simulink model "Copy_of_MPC_control"  (R2018a)
settings: Solver=FixedStepAuto  StartTime=0  StopTime=Tend  FixedStep=0.001  RelTol=5e-3
model workspace (MAT data in the model file):
  A_mu = 10
  B_reff = 8.386
  Cz = 7766.25
  DCT_Param : struct (value not decoded)
  D_reff = 0.25826
  Downshift_Speeds = [9.5625 12.9375 16.3125 19.6875 23.0625 26.4375 29.8125 33.1875 36.5625 39.9375 43.3125 46.6875 ... (28 elements, 4x7)]
  Pedal_Positions = [0.1 0.4 0.5 0.9]
  SUS : struct (value not decoded)
  Upshift_Speeds = [12.9375 16.3125 19.6875 33 26.4375 29.8125 33.1875 52.5 39.9375 43.3125 46.6875 77.25 ... (28 elements, 4x7)]
  VEH : struct (value not decoded)
  V_o = 16.7
  V_xlow = 1
  WH : struct (value not decoded)
  a = 1.4
  alpha_max = 1.5
  alpha_min = -1.5
  b = 1.8
  c_zo = 209651
  epsilon = 0.1
  h = 0.134
  path : struct (value not decoded)
  pio = 220000
  q_Fcx = 0
  q_Fz2 = 15.4
  q_Fzy = 0
  q_reo = 0.9974
  q_sx1 = -0.007764
  q_sx10 = 0.2824
  q_sx11 = 5.349
  q_sx12 = 0
  q_sx13 = 0
  q_sx14 = 0
  q_sx2 = 1.1915
  q_sx3 = 0.013948
  q_sx4 = 4.912
  q_sx5 = 1.02
  q_sx6 = 22.83
  q_sx7 = 0.7104
  q_sx8 = -0.023393
  q_sx9 = 0.6581
  q_sy1 = 0.00702
  q_sy2 = 0
  q_sy3 = 0.001515
  q_sy4 = 8.514e-05
  q_sy5 = 0
  q_sy6 = 0
  q_sy7 = 0.9008
  q_sy8 = -0.4089
  q_v1 = 0.0007742
  q_v2 = 0.04667
  r_Bx1 = 12.531
  r_Bx2 = 9.532
  r_Bx3 = 0
  r_By1 = 10.615
  r_By2 = 7.705
  r_By3 = 3.433e-06
  r_By4 = 0
  r_Cx1 = 1.019
  r_Cy1 = 1.0585
  r_Ex1 = -0.4487
  r_Ex2 = -0.4726
  r_Ey1 = 0.3132
  r_Ey2 = 7.63e-06
  r_Hx1 = 0.0002374
  r_Hy1 = 0.011646
  r_Hy2 = 7.63e-06
  r_Vy1 = 0.05654
  r_Vy2 = 7.63e-06
  r_Vy3 = 0
  r_Vy4 = 99.9
  r_Vy5 = 2
  r_Vy6 = 15.814
  r_o = 0.3135
  vehWidth = 2
  w = 1
symbols that are objects in the model workspace (value not decoded): VEH
undefined symbols (not defined in the file): C_Brake, C_Final, C_Front, C_Front_1, C_Front_2, C_Middle, C_out_Brake, C_out_Final, C_out_Front, C_out_Front_1, C_out_Front_2, C_out_Middle, Co, Cok_Brake, Cok_Final, Cok_Front_1, Cok_Front_2, Cok_Middle, Cso, D_out_Brake, D_out_Final, D_out_Front, D_out_Front_1, D_out_Front_2, D_out_Middle, Earlytochange, Earlytochange2, F, F_Brake, F_Final, F_Front, F_Front_1, F_Front_2, F_Middle, Fs, G_Brake, G_Final, G_Front_1, G_Front_2, G_Middle, G_sys_Brake, G_sys_Final, G_sys_Front, G_sys_Front_1, G_sys_Front_2, G_sys_Middle, Gd, Gd_Brake, Gd_Final, Gd_Front, Gd_Front_1, Gd_Front_2, Gd_Middle, Go, Gsd, Gso, H_Brake, H_Final, H_Front_1, H_Front_2 ... (+60)
libraries: simulink x10, sim3dlib x4, autolibutils x2, vehdynlibviscommon x2
(part 3 of 8)

== system Copy_of_MPC_control/all_system/Visualization1 ==
  note: Driver Commands
  note: Vehicle Response
  Cntrl : Inport
  VehFdbk : Inport  Port=2
  3D Engine : Subsystem  Variant=on  OverrideUsingVariant=0  mask(3D Engine){engine3D=Disabled, SceneDesc=Straight road, dt3D=.03}
      mask prompts: engine3D "3D Engine"; SceneDesc "Scene Description:"; dt3D "Engine frame rate, dt3D [s]:"
      mask help: This subsystem contains the interface blocks which permit the display of the vehicle in 3D virtual environment. Enable it to view the simulation progress, disable it to inhibit the display.
      mask init: same as Copy_of_MPC_control/Visualization/3D Engine
      settings: AttributesFormatString=%<engine3D>
      mask Help: eval('vdynblkshelp(''vdynblksscenecameraray'')');
      mask TypeOptions engine3D: Enabled | Disabled
      mask Callback engine3D:
      | switch get_param(gcb,'engine3D')
      |     case 'Disabled'
      |         set_param(gcb,'OverrideUsingVariant','0')
      |     case 'Enabled'
      |        set_param(gcb,'OverrideUsingVariant','1')
      |     otherwise
      |        set_param(gcb,'OverrideUsingVariant','0')
      | end
      mask TypeOptions SceneDesc:
      | 3D Engine/Simulation 3D Engine
      | 1/SceneDesc
      mask Display: disp('3D Engine')
  Acceleration Cmd : Subsystem  DialogController=hmiCreateDDGDialog  IsWebBlock=on  mask(MWDashboardBlock){webBlockId=2ec56b20-76c2-4aac-ab3d-2dd24ca42fe8, webBlockType=lineargauge, ShowInLibBrowser=on, ShowInitialText=on, HMISrcModelName=MPC_control}
      mask prompts: webBlockId "WebBlock Id"; webBlockType "WebBlock Type"; HMISrcModelName "Source Model"
      mask help: SimulinkHMI:dialogs:LinearGaugeDialogDesc
      mask Help: helpview([docroot '/mapfiles/simulink.map'], 'hmi_linear_gauge')
      mask Display:
      | if strcmp(get_param(bdroot(gcb),'BlockDiagramType'), 'library')
      |     image([(matlabroot) '/toolbox/simulink/hmi/icons/LinearGauge.png']);
      | end
  Brake Cmd : Subsystem  DialogController=hmiCreateDDGDialog  IsWebBlock=on  mask(MWDashboardBlock){webBlockId=d9917a9d-f04e-4f5f-9d8a-619b2f9adbbc, webBlockType=lineargauge, ShowInLibBrowser=on, ShowInitialText=on, HMISrcModelName=MPC_control}
      mask prompts: webBlockId "WebBlock Id"; webBlockType "WebBlock Type"; HMISrcModelName "Source Model"
      mask help: SimulinkHMI:dialogs:LinearGaugeDialogDesc
      mask Help: helpview([docroot '/mapfiles/simulink.map'], 'hmi_linear_gauge')
      mask Display:
      | if strcmp(get_param(bdroot(gcb),'BlockDiagramType'), 'library')
      |     image([(matlabroot) '/toolbox/simulink/hmi/icons/LinearGauge.png']);
      | end
  Bus Selector : BusSelector  OutputSignals=Driveline.EngSpd,Body.xdot,Body.ay
  Bus Selector2 : BusSelector  OutputSignals=Accel,Brake,Steer
  Bus Selector3 : BusSelector  OutputSignals=Body.r
  Engine Tach [rpm] : Subsystem  DialogController=hmiCreateDDGDialog  IsWebBlock=on  mask(MWDashboardBlock){webBlockId=b43bb858-1bc3-4216-8222-68d06605e534, webBlockType=circulargauge, ShowInLibBrowser=on, ShowInitialText=on, HMISrcModelName=MPC_control}
      mask prompts: webBlockId "WebBlock Id"; webBlockType "WebBlock Type"; HMISrcModelName "Source Model"
      mask help: SimulinkHMI:dialogs:CircularGaugeDialogDesc
      mask Help: helpview([docroot '/mapfiles/simulink.map'], 'hmi_gauge')
      mask Display:
      | if strcmp(get_param(bdroot(gcb),'BlockDiagramType'), 'library')
      |     image([(matlabroot) '/toolbox/simulink/hmi/icons/CircularGauge.png']);
      | end
  Handwheel Angle [deg] : Subsystem  DialogController=hmiCreateDDGDialog  IsWebBlock=on  mask(MWDashboardBlock){webBlockId=4efaf655-7637-4550-9856-9a687d94287b, webBlockType=semicirculargauge, ShowInLibBrowser=on, ShowInitialText=on, HMISrcModelName=MPC_control}
      mask prompts: webBlockId "WebBlock Id"; webBlockType "WebBlock Type"; HMISrcModelName "Source Model"
      mask help: SimulinkHMI:dialogs:SemicircularGaugeDialogDesc
      mask Help: helpview([docroot '/mapfiles/simulink.map'], 'hmi_half_gauge')
      mask Display:
      | if strcmp(get_param(bdroot(gcb),'BlockDiagramType'), 'library')
      |     image([(matlabroot) '/toolbox/simulink/hmi/icons/SemicircularGauge.png']);
      | end
  Lateral Acceleration [g] : Subsystem  DialogController=hmiCreateDDGDialog  IsWebBlock=on  mask(MWDashboardBlock){webBlockId=4c84f06f-3c50-4c9f-a814-1d904b0076de, webBlockType=semicirculargauge, ShowInLibBrowser=on, ShowInitialText=on, HMISrcModelName=MPC_control}
      mask prompts: webBlockId "WebBlock Id"; webBlockType "WebBlock Type"; HMISrcModelName "Source Model"
      mask help: SimulinkHMI:dialogs:SemicircularGaugeDialogDesc
      mask Help: helpview([docroot '/mapfiles/simulink.map'], 'hmi_half_gauge')
      mask Display:
      | if strcmp(get_param(bdroot(gcb),'BlockDiagramType'), 'library')
      |     image([(matlabroot) '/toolbox/simulink/hmi/icons/SemicircularGauge.png']);
      | end
  Rate Transition1 : RateTransition
  Rate Transition2 : RateTransition
  Signal Specification : SignalSpecification  Unit=deg
  Signal Specification1 : SignalSpecification  Unit=mph
  Signal Specification2 : SignalSpecification  Unit=deg/s
  Signal Specification3 : SignalSpecification  Unit=rpm
  Speed [mph] : Subsystem  DialogController=hmiCreateDDGDialog  IsWebBlock=on  mask(MWDashboardBlock){webBlockId=6d425e54-616c-4430-b762-4652b407af79, webBlockType=circulargauge, ShowInLibBrowser=on, ShowInitialText=on, HMISrcModelName=MPC_control}
      mask prompts: webBlockId "WebBlock Id"; webBlockType "WebBlock Type"; HMISrcModelName "Source Model"
      mask help: SimulinkHMI:dialogs:CircularGaugeDialogDesc
      mask Help: helpview([docroot '/mapfiles/simulink.map'], 'hmi_gauge')
      mask Display:
      | if strcmp(get_param(bdroot(gcb),'BlockDiagramType'), 'library')
      |     image([(matlabroot) '/toolbox/simulink/hmi/icons/CircularGauge.png']);
      | end
  Start Steering Command : LampBlock  WebBlockId=9740  LabelPosition=Hide
  Steer vs Ay : simulink/Sinks/XY Graph  Commented=on  xmin=-300  xmax=300  ymin=-1.5  ymax=1.5  st=.1
  "Steer, Velocity, Lat Accel" : Scope  NumInputPorts=3
  Terminator{,1..3} (4 alike) : Terminator
  Unit Conversion{1..4} (4 alike) : UnitConversion
  Vehicle XY Plotter : Subsystem  mask(Vehicle XY Plotter){a=VEH.FrontAxlePositionfromCG, b=VEH.RearAxlePositionfromCG, w=VEH.TrackWidth, bufferSize=1024, pltDT=0.1}
      mask prompts: a "Distance to front axle from CG, a [m]:"; b "Distance to rear axle from CG, b [m]:"; w "Track width, w [m]:"; bufferSize "Path buffer sampe size, bufferSize []:"; pltDT "Plot update rate, pltDT [s]:"
      mask help: This block will display a MATLAB figure which indicates the vehicle path, current position and heading velocity.
      mask TypeOptions a: Vehicle XY Plotter/a
      mask TypeOptions b: Vehicle XY Plotter/b
      mask TypeOptions w: Vehicle XY Plotter/w
      mask TypeOptions bufferSize: Vehicle XY Plotter/bufferSize
  Yaw Rate and Steer : Scope  NumInputPorts=2
  wires:
  Unit Conversion3/1 -> Signal Specification2/1
  Bus Selector3/1 -> Unit Conversion3/1  "<r>"
  Signal Specification2/1 -> Yaw Rate and Steer/1
  Unit Conversion4/1 -> Signal Specification3/1
  Signal Specification3/1 -> Terminator3/1  "Engine_rpm"
  Signal Specification/1 -> Yaw Rate and Steer/2, Rate Transition1/1, "Steer, Velocity, Lat Accel"/1  "SteerAngle"
  Bus Selector2/3 -> Unit Conversion2/1  "<Steer>"
  Signal Specification1/1 -> Terminator/1  "xdot_mph"
  Unit Conversion1/1 -> Signal Specification1/1
  Bus Selector/3 -> Rate Transition2/1, "Steer, Velocity, Lat Accel"/3  "<ay>"
  Bus Selector2/1 -> Terminator1/1  "<Accel>"
  Rate Transition1/1 -> Steer vs Ay/1
  Unit Conversion2/1 -> Signal Specification/1
  Bus Selector/2 -> "Steer, Velocity, Lat Accel"/2, Unit Conversion1/1  "<xdot>"
  VehFdbk/1 -> Bus Selector3/1, Bus Selector/1, Vehicle XY Plotter/1(VehFdbk), 3D Engine/1(VehFdbk)  "VehFdbk"
  Cntrl/1 -> Bus Selector2/1
  Rate Transition2/1 -> Steer vs Ay/2
  Bus Selector/1 -> Unit Conversion4/1  "<EngSpd>"
  Bus Selector2/2 -> Terminator2/1  "<Brake>"

== system Copy_of_MPC_control/all_system/YV_update_Np1 ==
  XY_sim : Inport
  Velocity_sim : Inport  Port=2
  Heading_sim : Inport  Port=3
  From Workspace1 : FromWorkspace  VariableName=T_sim  SampleTime=Ts
  From Workspace3 : FromWorkspace  VariableName=XY_Ref_Upd  SampleTime=Ts
  MATLAB Function2 : MATLAB Function  TreatAsAtomicUnit=on  SystemSampleTime=Ts
  Unit Delay1 : UnitDelay  SampleTime=Ts
  Unit Delay4 : UnitDelay  SampleTime=Ts
  Unit Delay5 : UnitDelay  SampleTime=Ts
  Velocity : Outport
  Heading angle : Outport  Port=2
  wires:
  MATLAB Function2/1(Velocity_updated) -> Velocity/1
  From Workspace3/1 -> MATLAB Function2/1(XY_ref)
  MATLAB Function2/2(Heading_updated) -> Heading angle/1
  From Workspace1/1 -> MATLAB Function2/8(Tsim)
  XY_sim/1 -> Unit Delay1/1, MATLAB Function2/2(XY_sim)
  Velocity_sim/1 -> MATLAB Function2/4(Velocity_sim), Unit Delay5/1
  Heading_sim/1 -> MATLAB Function2/6(Yaw_sim), Unit Delay4/1
  Unit Delay1/1 -> MATLAB Function2/3(LastXY_sim)
  Unit Delay5/1 -> MATLAB Function2/5(LastVelocity_sim)
  Unit Delay4/1 -> MATLAB Function2/7(LastYaw_sim)

== system Copy_of_MPC_control/observer/observer_1 ==
  r(k-1) : Inport
  U_delay : Inport  Port=2
  Y : Inport  Port=3
  Y_overlap : Inport  Port=4
  U : Inport  Port=5
  U_overlap : Inport  Port=6
  Cok_Front_1 : Gain  Gain=Cok_Front_1  Multiplication=Matrix(K*u) (u vector)
  Delay : Delay  DelayLength=1  InitialConditionSource=Input port  InitialCondition=0  ExternalReset=Rising  SampleTime=Ts
      settings: InputPortMap=u0,r5,p4
  Delay1 : Delay  DelayLength=1  InitialConditionSource=Input port  InitialCondition=0  ExternalReset=Rising  SampleTime=Ts
      settings: InputPortMap=u0,r5,p4
  From Workspace2 : FromWorkspace  VariableName=select_overlap  SampleTime=Ts
  Gd_Front_1 : Gain  Gain=Gd_Front_1  Multiplication=Matrix(K*u) (u vector)
  Hd_Front_1 : Gain  Gain=Hd_Front_1  Multiplication=Matrix(K*u) (u vector)
  Ld_Front_1 : Gain  Gain=Ld_Front_1  Multiplication=Matrix(K*u) (u vector)
  Ld_Front_1* : Gain  Gain=Ld_Front_1  Multiplication=Matrix(K*u) (u vector)
  Sum4 : Sum  Inputs=+++
  Switch1 : Switch  Threshold=1
  Switch2 : Switch  Threshold=1
  gate : MATLAB Function  TreatAsAtomicUnit=on
  xhat : Outport
  wires:
  Hd_Front_1/1 -> Sum4/2
  Ld_Front_1/1 -> Sum4/1
  Delay1/1 -> Hd_Front_1/1
  U_overlap/1 -> Switch2/1
  Gd_Front_1/1 -> Sum4/3
  Switch1/1 -> Ld_Front_1/1
  Switch2/1 -> Delay1/1
  Ld_Front_1*/1 -> Delay/3
  Sum4/1 -> xhat/1, Delay/1, Cok_Front_1/1  "xhat"
  Delay/1 -> Gd_Front_1/1
  Y_overlap/1 -> Switch1/1
  U/1 -> Switch2/3
  Y/1 -> Switch1/3
  U_delay/1 -> Delay1/3
  gate/1(state) -> Delay/2, Delay1/2, Switch2/2, Switch1/2
  From Workspace2/1 -> gate/1(select_overlap)
  r(k-1)/1 -> Ld_Front_1*/1

== system Copy_of_MPC_control/observer/observer_2 ==
  r(k-1) : Inport
  U_delay : Inport  Port=2
  Y : Inport  Port=3
  Y_overlap : Inport  Port=4
  U : Inport  Port=5
  U_overlap : Inport  Port=6
  Cok_Front_2 : Gain  Gain=Cok_Front_2  Multiplication=Matrix(K*u) (u vector)
  Delay : Delay  DelayLength=1  InitialConditionSource=Input port  InitialCondition=0  ExternalReset=Rising  SampleTime=Ts
      settings: InputPortMap=u0,r5,p4
  Delay1 : Delay  DelayLength=1  InitialConditionSource=Input port  InitialCondition=0  ExternalReset=Rising  SampleTime=Ts
      settings: InputPortMap=u0,r5,p4
  From Workspace2 : FromWorkspace  VariableName=select_overlap  SampleTime=Ts
  Gd_Front_2 : Gain  Gain=Gd_Front_2  Multiplication=Matrix(K*u) (u vector)
  Hd_Front_2 : Gain  Gain=Hd_Front_2  Multiplication=Matrix(K*u) (u vector)
  Ld_Front_2 : Gain  Gain=Ld_Front_2  Multiplication=Matrix(K*u) (u vector)
  Ld_Front_2* : Gain  Gain=Ld_Front_2  Multiplication=Matrix(K*u) (u vector)
  Sum4 : Sum  Inputs=+++
  Switch1 : Switch  Threshold=1
  Switch2 : Switch  Threshold=1
  gate : MATLAB Function  TreatAsAtomicUnit=on
  xhat : Outport
  wires:
  Hd_Front_2/1 -> Sum4/2
  Ld_Front_2/1 -> Sum4/1
  Delay1/1 -> Hd_Front_2/1
  U_overlap/1 -> Switch2/1
  Gd_Front_2/1 -> Sum4/3
  Switch1/1 -> Ld_Front_2/1
  Switch2/1 -> Delay1/1
  Ld_Front_2*/1 -> Delay/3
  Sum4/1 -> xhat/1, Delay/1, Cok_Front_2/1  "xhat"
  Delay/1 -> Gd_Front_2/1
  Y_overlap/1 -> Switch1/1
  U/1 -> Switch2/3
  Y/1 -> Switch1/3
  U_delay/1 -> Delay1/3
  gate/1(state) -> Delay/2, Delay1/2, Switch2/2, Switch1/2
  From Workspace2/1 -> gate/1(select_overlap)
  r(k-1)/1 -> Ld_Front_2*/1

== system Copy_of_MPC_control/observer/observer_3 ==
  r(k-1) : Inport
  U_delay : Inport  Port=2
  Y : Inport  Port=3
  Y_overlap : Inport  Port=4
  U : Inport  Port=5
  U_overlap : Inport  Port=6
  Cok_Middle : Gain  Gain=Cok_Middle  Multiplication=Matrix(K*u) (u vector)
  Delay : Delay  DelayLength=1  InitialConditionSource=Input port  InitialCondition=0  ExternalReset=Rising  SampleTime=Ts
      settings: InputPortMap=u0,r5,p4
  Delay1 : Delay  DelayLength=1  InitialConditionSource=Input port  InitialCondition=0  ExternalReset=Rising  SampleTime=Ts
      settings: InputPortMap=u0,r5,p4
  From Workspace2 : FromWorkspace  VariableName=select_overlap  SampleTime=Ts
  Gd_Middle : Gain  Gain=Gd_Middle  Multiplication=Matrix(K*u) (u vector)
  Hd_Middle : Gain  Gain=Hd_Middle  Multiplication=Matrix(K*u) (u vector)
  Ld_Middle : Gain  Gain=Ld_Middle  Multiplication=Matrix(K*u) (u vector)
  Ld_Middle* : Gain  Gain=Ld_Middle  Multiplication=Matrix(K*u) (u vector)
  Sum4 : Sum  Inputs=+++
  Switch1 : Switch  Threshold=1
  Switch2 : Switch  Threshold=1
  gate : MATLAB Function  TreatAsAtomicUnit=on
  xhat : Outport
  wires:
  Hd_Middle/1 -> Sum4/2
  Ld_Middle/1 -> Sum4/1
  Delay1/1 -> Hd_Middle/1
  U_overlap/1 -> Switch2/1
  Gd_Middle/1 -> Sum4/3
  Switch1/1 -> Ld_Middle/1
  Switch2/1 -> Delay1/1
  Ld_Middle*/1 -> Delay/3
  Sum4/1 -> xhat/1, Delay/1, Cok_Middle/1  "xhat"
  Delay/1 -> Gd_Middle/1
  Y_overlap/1 -> Switch1/1
  U/1 -> Switch2/3
  Y/1 -> Switch1/3
  U_delay/1 -> Delay1/3
  gate/1(state) -> Delay/2, Delay1/2, Switch2/2, Switch1/2
  From Workspace2/1 -> gate/1(select_overlap)
  r(k-1)/1 -> Ld_Middle*/1

== system Copy_of_MPC_control/observer/observer_4 ==
  r(k-1) : Inport
  U_delay : Inport  Port=2
  Y : Inport  Port=3
  Y_overlap : Inport  Port=4
  U : Inport  Port=5
  U_overlap : Inport  Port=6
  Cok_Final : Gain  Gain=Cok_Final  Multiplication=Matrix(K*u) (u vector)
  Delay : Delay  DelayLength=1  InitialConditionSource=Input port  InitialCondition=0  ExternalReset=Rising  SampleTime=Ts
      settings: InputPortMap=u0,r5,p4
  Delay1 : Delay  DelayLength=1  InitialConditionSource=Input port  InitialCondition=0  ExternalReset=Rising  SampleTime=Ts
      settings: InputPortMap=u0,r5,p4
  From Workspace2 : FromWorkspace  VariableName=select_overlap  SampleTime=Ts
  Gd_Final : Gain  Gain=Gd_Final  Multiplication=Matrix(K*u) (u vector)
  Hd_Final : Gain  Gain=Hd_Final  Multiplication=Matrix(K*u) (u vector)
  Ld_Final : Gain  Gain=Ld_Final  Multiplication=Matrix(K*u) (u vector)
  Ld_Final* : Gain  Gain=Ld_Final  Multiplication=Matrix(K*u) (u vector)
  Sum4 : Sum  Inputs=+++
  Switch1 : Switch  Threshold=1
  Switch2 : Switch  Threshold=1
  gate : MATLAB Function  TreatAsAtomicUnit=on
  xhat : Outport
  wires:
  Hd_Final/1 -> Sum4/2
  Ld_Final/1 -> Sum4/1
  Delay1/1 -> Hd_Final/1
  U_overlap/1 -> Switch2/1
  Gd_Final/1 -> Sum4/3
  Switch1/1 -> Ld_Final/1
  Switch2/1 -> Delay1/1
  Ld_Final*/1 -> Delay/3
  Sum4/1 -> xhat/1, Delay/1, Cok_Final/1  "xhat"
  Delay/1 -> Gd_Final/1
  Y_overlap/1 -> Switch1/1
  U/1 -> Switch2/3
  Y/1 -> Switch1/3
  U_delay/1 -> Delay1/3
  gate/1(state) -> Delay/2, Delay1/2, Switch2/2, Switch1/2
  From Workspace2/1 -> gate/1(select_overlap)
  r(k-1)/1 -> Ld_Final*/1

== system Copy_of_MPC_control/observer/observer_5 ==
  r(k-1) : Inport
  U_delay : Inport  Port=2
  Y : Inport  Port=3
  Y_overlap : Inport  Port=4
  U : Inport  Port=5
  U_overlap : Inport  Port=6
  Cok_Brake : Gain  Gain=Cok_Brake  Multiplication=Matrix(K*u) (u vector)
  Delay : Delay  DelayLength=1  InitialConditionSource=Input port  InitialCondition=0  ExternalReset=Rising  SampleTime=Ts
      settings: InputPortMap=u0,r5,p4
  Delay1 : Delay  DelayLength=1  InitialConditionSource=Input port  InitialCondition=0  ExternalReset=Rising  SampleTime=Ts
      settings: InputPortMap=u0,r5,p4
  From Workspace2 : FromWorkspace  VariableName=select_overlap  SampleTime=Ts
  Gd_Brake : Gain  Gain=Gd_Brake  Multiplication=Matrix(K*u) (u vector)
  Hd_Brake : Gain  Gain=Hd_Brake  Multiplication=Matrix(K*u) (u vector)
  Ld_Brake : Gain  Gain=Ld_Brake  Multiplication=Matrix(K*u) (u vector)
  Ld_Brake* : Gain  Gain=Ld_Brake  Multiplication=Matrix(K*u) (u vector)
  Sum4 : Sum  Inputs=+++
  Switch1 : Switch  Threshold=1
  Switch2 : Switch  Threshold=1
  gate : MATLAB Function  TreatAsAtomicUnit=on
  xhat : Outport
  wires:
  Hd_Brake/1 -> Sum4/2
  Ld_Brake/1 -> Sum4/1
  Delay1/1 -> Hd_Brake/1
  U_overlap/1 -> Switch2/1
  Gd_Brake/1 -> Sum4/3
  Switch1/1 -> Ld_Brake/1
  Switch2/1 -> Delay1/1
  Ld_Brake*/1 -> Delay/3
  Sum4/1 -> xhat/1, Delay/1, Cok_Brake/1  "xhat"
  Delay/1 -> Gd_Brake/1
  Y_overlap/1 -> Switch1/1
  U/1 -> Switch2/3
  Y/1 -> Switch1/3
  U_delay/1 -> Delay1/3
  gate/1(state) -> Delay/2, Delay1/2, Switch2/2, Switch1/2
  From Workspace2/1 -> gate/1(select_overlap)
  r(k-1)/1 -> Ld_Brake*/1

== system Copy_of_MPC_control/observer/simulator_1 ==
  r(k) : Inport
  r(k-1) : Inport  Port=2
  Initial position : Inport  Port=3
  Initial Velocities : Inport  Port=4
  Initial HeadingAngles : Inport  Port=5
  U_delay : Inport  Port=6
  xhat : Inport  Port=7
  C_Front_1 : Gain  Gain=C_Front_1  Multiplication=Matrix(K*u) (u vector)
  C_Front_1* : Gain  Gain=C_Front_1  Multiplication=Matrix(K*u) (u vector)
  C_out_Front_1 : Gain  Gain=C_out_Front_1  Multiplication=Matrix(K*u) (u vector)
  D_out_Front_1 : Gain  Gain=D_out_Front_1  Multiplication=Matrix(K*u) (u vector)
  Demux : Demux  Outputs=2
  From Workspace2 : FromWorkspace  VariableName=select_overlap  SampleTime=Ts
  G_Front_1 : Gain  Gain=G_Front_1  Multiplication=Matrix(K*u) (u vector)
  G_sys_Front_1 : Gain  Gain=G_sys_Front_1  Multiplication=Matrix(K*u) (u vector)
  H_Front_1 : Gain  Gain=H_Front_1  Multiplication=Matrix(K*u) (u vector)
  H_sys_Front_1 : Gain  Gain=H_sys_Front_1  Multiplication=Matrix(K*u) (u vector)
  Ld_Front_1 : Gain  Gain=Ld_Front_1  Multiplication=Matrix(K*u) (u vector)
  Ld_Front_1* : Gain  Gain=Ld_Front_1  Multiplication=Matrix(K*u) (u vector)
  Ld_Front_1** : Gain  Gain=Ld_Front_1  Multiplication=Matrix(K*u) (u vector)
  Mpc_Simulator_Middle : Subsystem
  Resettable Delay : Delay  DelayLength=1  InitialConditionSource=Input port  ExternalReset=Rising  SampleTime=Ts
      settings: InputPortMap=u0,r5,p4
  Resettable Delay1 : Delay  DelayLength=1  InitialConditionSource=Input port  ExternalReset=Rising  SampleTime=Ts
      settings: InputPortMap=u0,r5,p4
  Resettable Delay2 : Delay  DelayLength=1  InitialConditionSource=Input port  ExternalReset=Rising  SampleTime=Ts
      settings: InputPortMap=u0,r5,p4
  Sum1 : Sum  Inputs=+++
  Sum2 : Sum  Inputs=+++
  Sum6 : Sum
  Sum7 : Sum  Inputs=-+
  VH2P : Subsystem
  YV_update_Np : Subsystem  TreatAsAtomicUnit=on
  gate : MATLAB Function  TreatAsAtomicUnit=on
  Y_overlap : Outport
  U_overlap : Outport  Port=2
  wires:
  Initial position/1 -> VH2P/3(Initial position)
  Sum2/1 -> Resettable Delay/1
  Demux/2 -> YV_update_Np/3(Heading_sim), VH2P/2(HeadingAngles)
  Ld_Front_1/1 -> Sum2/1
  Sum7/1 -> Ld_Front_1/1
  Mpc_Simulator_Middle/2(r) -> Sum7/2
  C_out_Front_1/1 -> Sum1/3
  C_Front_1*/1 -> Sum7/1
  Mpc_Simulator_Middle/1(U) -> Resettable Delay1/1, H_sys_Front_1/1, H_Front_1/1, U_overlap/1
  H_sys_Front_1/1 -> Sum2/2
  G_sys_Front_1/1 -> Sum2/3
  Resettable Delay2/1 -> C_out_Front_1/1
  VH2P/1(Position) -> YV_update_Np/1(XY_sim)
  Demux/1 -> VH2P/1(Velocities), YV_update_Np/2(Velocity_sim)
  Resettable Delay/1 -> G_sys_Front_1/1, Resettable Delay2/1, G_Front_1/1, C_Front_1/1
  H_Front_1/1 -> Sum6/1
  Sum1/1 -> Demux/1, Y_overlap/1
  Sum6/1 -> C_Front_1*/1
  D_out_Front_1/1 -> Sum1/2
  Resettable Delay1/1 -> D_out_Front_1/1
  C_Front_1/1 -> Sum1/1
  YV_update_Np/2(Heading_updated) -> Mpc_Simulator_Middle/2(Heading_updated)
  xhat/1 -> Mpc_Simulator_Middle/3(Xhat)
  YV_update_Np/1(Velocity_updated) -> Mpc_Simulator_Middle/1(Velocity_updated)
  r(k)/1 -> Ld_Front_1*/1
  Ld_Front_1*/1 -> Resettable Delay/3
  U_delay/1 -> Resettable Delay1/3
  r(k-1)/1 -> Ld_Front_1**/1
  Ld_Front_1**/1 -> Resettable Delay2/3
  Initial Velocities/1 -> VH2P/4(Iintial Velocities)
  Initial HeadingAngles/1 -> VH2P/5(Iintial HeadingAngles)
  From Workspace2/1 -> gate/1(select_overlap)
  gate/1(state) -> Resettable Delay/2, Resettable Delay1/2, Resettable Delay2/2
  G_Front_1/1 -> Sum6/2

== system Copy_of_MPC_control/observer/simulator_2 ==
  r(k) : Inport
  r(k-1) : Inport  Port=2
  Initial position : Inport  Port=3
  Initial Velocities : Inport  Port=4
  Initial HeadingAngles : Inport  Port=5
  U_delay : Inport  Port=6
  xhat : Inport  Port=7
  C_Front_2 : Gain  Gain=C_Front_2  Multiplication=Matrix(K*u) (u vector)
  C_Front_2* : Gain  Gain=C_Front_2  Multiplication=Matrix(K*u) (u vector)
  C_out_Front_2 : Gain  Gain=C_out_Front_2  Multiplication=Matrix(K*u) (u vector)
  D_out_Front_2 : Gain  Gain=D_out_Front_2  Multiplication=Matrix(K*u) (u vector)
  Demux : Demux  Outputs=2
  From Workspace2 : FromWorkspace  VariableName=select_overlap  SampleTime=Ts
  G_Front_2 : Gain  Gain=G_Front_2  Multiplication=Matrix(K*u) (u vector)
  G_sys_Front_2 : Gain  Gain=G_sys_Front_2  Multiplication=Matrix(K*u) (u vector)
  H_Front_2 : Gain  Gain=H_Front_2  Multiplication=Matrix(K*u) (u vector)
  H_sys_Front_2 : Gain  Gain=H_sys_Front_2  Multiplication=Matrix(K*u) (u vector)
  Ld_Front_2 : Gain  Gain=Ld_Front_2  Multiplication=Matrix(K*u) (u vector)
  Ld_Front_2* : Gain  Gain=Ld_Front_2  Multiplication=Matrix(K*u) (u vector)
  Ld_Front_2** : Gain  Gain=Ld_Front_2  Multiplication=Matrix(K*u) (u vector)
  Mpc_Simulator_Middle : Subsystem
  Resettable Delay : Delay  DelayLength=1  InitialConditionSource=Input port  ExternalReset=Rising  SampleTime=Ts
      settings: InputPortMap=u0,r5,p4
  Resettable Delay1 : Delay  DelayLength=1  InitialConditionSource=Input port  ExternalReset=Rising  SampleTime=Ts
      settings: InputPortMap=u0,r5,p4
  Resettable Delay2 : Delay  DelayLength=1  InitialConditionSource=Input port  ExternalReset=Rising  SampleTime=Ts
      settings: InputPortMap=u0,r5,p4
  Sum1 : Sum  Inputs=+++
  Sum2 : Sum  Inputs=+++
  Sum6 : Sum
  Sum7 : Sum  Inputs=-+
  VH2P : Subsystem
  YV_update_Np : Subsystem  TreatAsAtomicUnit=on
  gate : MATLAB Function  TreatAsAtomicUnit=on
  Y_overlap : Outport
  U_overlap : Outport  Port=2
  wires:
  Initial position/1 -> VH2P/3(Initial position)
  Sum2/1 -> Resettable Delay/1
  Demux/2 -> YV_update_Np/3(Heading_sim), VH2P/2(HeadingAngles)
  Ld_Front_2/1 -> Sum2/1
  Sum7/1 -> Ld_Front_2/1
  Mpc_Simulator_Middle/2(r) -> Sum7/2
  C_out_Front_2/1 -> Sum1/3
  C_Front_2*/1 -> Sum7/1
  Mpc_Simulator_Middle/1(U) -> Resettable Delay1/1, H_sys_Front_2/1, H_Front_2/1, U_overlap/1
  H_sys_Front_2/1 -> Sum2/2
  G_sys_Front_2/1 -> Sum2/3
  Resettable Delay2/1 -> C_out_Front_2/1
  VH2P/1(Position) -> YV_update_Np/1(XY_sim)
  Demux/1 -> VH2P/1(Velocities), YV_update_Np/2(Velocity_sim)
  Resettable Delay/1 -> G_sys_Front_2/1, Resettable Delay2/1, G_Front_2/1, C_Front_2/1
  H_Front_2/1 -> Sum6/1
  Sum1/1 -> Demux/1, Y_overlap/1
  Sum6/1 -> C_Front_2*/1
  D_out_Front_2/1 -> Sum1/2
  Resettable Delay1/1 -> D_out_Front_2/1
  C_Front_2/1 -> Sum1/1
  YV_update_Np/2(Heading_updated) -> Mpc_Simulator_Middle/2(Heading_updated)
  xhat/1 -> Mpc_Simulator_Middle/3(Xhat)
  YV_update_Np/1(Velocity_updated) -> Mpc_Simulator_Middle/1(Velocity_updated)
  r(k)/1 -> Ld_Front_2*/1
  Ld_Front_2*/1 -> Resettable Delay/3
  U_delay/1 -> Resettable Delay1/3
  r(k-1)/1 -> Ld_Front_2**/1
  Ld_Front_2**/1 -> Resettable Delay2/3
  Initial Velocities/1 -> VH2P/4(Iintial Velocities)
  Initial HeadingAngles/1 -> VH2P/5(Iintial HeadingAngles)
  From Workspace2/1 -> gate/1(select_overlap)
  gate/1(state) -> Resettable Delay/2, Resettable Delay1/2, Resettable Delay2/2
  G_Front_2/1 -> Sum6/2

== system Copy_of_MPC_control/observer/simulator_3 ==
  r(k) : Inport
  r(k-1) : Inport  Port=2
  Initial position : Inport  Port=3
  Initial Velocities : Inport  Port=4
  Initial HeadingAngles : Inport  Port=5
  U_delay : Inport  Port=6
  xhat : Inport  Port=7
  C_Middle : Gain  Gain=C_Middle  Multiplication=Matrix(K*u) (u vector)
  C_Middle* : Gain  Gain=C_Middle  Multiplication=Matrix(K*u) (u vector)
  C_out_Middle : Gain  Gain=C_out_Middle  Multiplication=Matrix(K*u) (u vector)
  D_out_Middle : Gain  Gain=D_out_Middle  Multiplication=Matrix(K*u) (u vector)
  Demux : Demux  Outputs=2
  From Workspace2 : FromWorkspace  VariableName=select_overlap  SampleTime=Ts
  G_Middle : Gain  Gain=G_Middle  Multiplication=Matrix(K*u) (u vector)
  G_sys_Middle : Gain  Gain=G_sys_Middle  Multiplication=Matrix(K*u) (u vector)
  H_Middle : Gain  Gain=H_Middle  Multiplication=Matrix(K*u) (u vector)
  H_sys_Middle : Gain  Gain=H_sys_Middle  Multiplication=Matrix(K*u) (u vector)
  Ld_Middle : Gain  Gain=Ld_Middle  Multiplication=Matrix(K*u) (u vector)
  Ld_Middle* : Gain  Gain=Ld_Middle  Multiplication=Matrix(K*u) (u vector)
  Ld_Middle** : Gain  Gain=Ld_Middle  Multiplication=Matrix(K*u) (u vector)
  Mpc_Simulator_Middle : Subsystem
  Resettable Delay : Delay  DelayLength=1  InitialConditionSource=Input port  ExternalReset=Rising  SampleTime=Ts
      settings: InputPortMap=u0,r5,p4
  Resettable Delay1 : Delay  DelayLength=1  InitialConditionSource=Input port  ExternalReset=Rising  SampleTime=Ts
      settings: InputPortMap=u0,r5,p4
  Resettable Delay2 : Delay  DelayLength=1  InitialConditionSource=Input port  ExternalReset=Rising  SampleTime=Ts
      settings: InputPortMap=u0,r5,p4
  Sum1 : Sum  Inputs=+++
  Sum2 : Sum  Inputs=+++
  Sum6 : Sum
  Sum7 : Sum  Inputs=-+
  VH2P : Subsystem
  YV_update_Np : Subsystem  TreatAsAtomicUnit=on
  gate : MATLAB Function  TreatAsAtomicUnit=on
  Y_overlap : Outport
  U_overlap : Outport  Port=2
  wires:
  Initial position/1 -> VH2P/3(Initial position)
  Sum2/1 -> Resettable Delay/1
  Demux/2 -> YV_update_Np/3(Heading_sim), VH2P/2(HeadingAngles)
  Ld_Middle/1 -> Sum2/1
  Sum7/1 -> Ld_Middle/1
  Mpc_Simulator_Middle/2(r) -> Sum7/2
  C_out_Middle/1 -> Sum1/3
  C_Middle*/1 -> Sum7/1
  Mpc_Simulator_Middle/1(U) -> Resettable Delay1/1, H_sys_Middle/1, H_Middle/1, U_overlap/1
  H_sys_Middle/1 -> Sum2/2
  G_sys_Middle/1 -> Sum2/3
  Resettable Delay2/1 -> C_out_Middle/1
  VH2P/1(Position) -> YV_update_Np/1(XY_sim)
  Demux/1 -> VH2P/1(Velocities), YV_update_Np/2(Velocity_sim)
  Resettable Delay/1 -> G_sys_Middle/1, Resettable Delay2/1, G_Middle/1, C_Middle/1
  H_Middle/1 -> Sum6/1
  Sum1/1 -> Demux/1, Y_overlap/1
  Sum6/1 -> C_Middle*/1
  D_out_Middle/1 -> Sum1/2
  Resettable Delay1/1 -> D_out_Middle/1
  C_Middle/1 -> Sum1/1
  YV_update_Np/2(Heading_updated) -> Mpc_Simulator_Middle/2(Heading_updated)
  xhat/1 -> Mpc_Simulator_Middle/3(Xhat)
  YV_update_Np/1(Velocity_updated) -> Mpc_Simulator_Middle/1(Velocity_updated)
  r(k)/1 -> Ld_Middle*/1
  Ld_Middle*/1 -> Resettable Delay/3
  U_delay/1 -> Resettable Delay1/3
  r(k-1)/1 -> Ld_Middle**/1
  Ld_Middle**/1 -> Resettable Delay2/3
  Initial Velocities/1 -> VH2P/4(Iintial Velocities)
  Initial HeadingAngles/1 -> VH2P/5(Iintial HeadingAngles)
  From Workspace2/1 -> gate/1(select_overlap)
  gate/1(state) -> Resettable Delay/2, Resettable Delay1/2, Resettable Delay2/2
  G_Middle/1 -> Sum6/2

== system Copy_of_MPC_control/observer/simulator_4 ==
  r(k) : Inport
  r(k-1) : Inport  Port=2
  Initial position : Inport  Port=3
  Initial Velocities : Inport  Port=4
  Initial HeadingAngles : Inport  Port=5
  U_delay : Inport  Port=6
  xhat : Inport  Port=7
  C_Final : Gain  Gain=C_Final  Multiplication=Matrix(K*u) (u vector)
  C_Final* : Gain  Gain=C_Final  Multiplication=Matrix(K*u) (u vector)
  C_out_Final : Gain  Gain=C_out_Final  Multiplication=Matrix(K*u) (u vector)
  D_out_Final : Gain  Gain=D_out_Final  Multiplication=Matrix(K*u) (u vector)
  Demux : Demux  Outputs=2
  From Workspace2 : FromWorkspace  VariableName=select_overlap  SampleTime=Ts
  G_Final : Gain  Gain=G_Final  Multiplication=Matrix(K*u) (u vector)
  G_sys_Final : Gain  Gain=G_sys_Final  Multiplication=Matrix(K*u) (u vector)
  H_Final : Gain  Gain=H_Final  Multiplication=Matrix(K*u) (u vector)
  H_sys_Final : Gain  Gain=H_sys_Final  Multiplication=Matrix(K*u) (u vector)
  Ld_Final : Gain  Gain=Ld_Final  Multiplication=Matrix(K*u) (u vector)
  Ld_Final* : Gain  Gain=Ld_Final  Multiplication=Matrix(K*u) (u vector)
  Ld_Final** : Gain  Gain=Ld_Final  Multiplication=Matrix(K*u) (u vector)
  Mpc_Simulator_Middle : Subsystem
  Resettable Delay : Delay  DelayLength=1  InitialConditionSource=Input port  ExternalReset=Rising  SampleTime=Ts
      settings: InputPortMap=u0,r5,p4
  Resettable Delay1 : Delay  DelayLength=1  InitialConditionSource=Input port  ExternalReset=Rising  SampleTime=Ts
      settings: InputPortMap=u0,r5,p4
  Resettable Delay2 : Delay  DelayLength=1  InitialConditionSource=Input port  ExternalReset=Rising  SampleTime=Ts
      settings: InputPortMap=u0,r5,p4
  Sum1 : Sum  Inputs=+++
  Sum2 : Sum  Inputs=+++
  Sum6 : Sum
  Sum7 : Sum  Inputs=-+
  VH2P : Subsystem
  YV_update_Np : Subsystem  TreatAsAtomicUnit=on
  gate : MATLAB Function  TreatAsAtomicUnit=on
  Y_overlap : Outport
  U_overlap : Outport  Port=2
  wires:
  Initial position/1 -> VH2P/3(Initial position)
  Sum2/1 -> Resettable Delay/1
  Demux/2 -> YV_update_Np/3(Heading_sim), VH2P/2(HeadingAngles)
  Ld_Final/1 -> Sum2/1
  Sum7/1 -> Ld_Final/1
  Mpc_Simulator_Middle/2(r) -> Sum7/2
  C_out_Final/1 -> Sum1/3
  C_Final*/1 -> Sum7/1
  Mpc_Simulator_Middle/1(U) -> Resettable Delay1/1, H_sys_Final/1, H_Final/1, U_overlap/1
  H_sys_Final/1 -> Sum2/2
  G_sys_Final/1 -> Sum2/3
  Resettable Delay2/1 -> C_out_Final/1
  VH2P/1(Position) -> YV_update_Np/1(XY_sim)
  Demux/1 -> VH2P/1(Velocities), YV_update_Np/2(Velocity_sim)
  Resettable Delay/1 -> G_sys_Final/1, Resettable Delay2/1, G_Final/1, C_Final/1
  H_Final/1 -> Sum6/1
  Sum1/1 -> Demux/1, Y_overlap/1
  Sum6/1 -> C_Final*/1
  D_out_Final/1 -> Sum1/2
  Resettable Delay1/1 -> D_out_Final/1
  C_Final/1 -> Sum1/1
  YV_update_Np/2(Heading_updated) -> Mpc_Simulator_Middle/2(Heading_updated)
  xhat/1 -> Mpc_Simulator_Middle/3(Xhat)
  YV_update_Np/1(Velocity_updated) -> Mpc_Simulator_Middle/1(Velocity_updated)
  r(k)/1 -> Ld_Final*/1
  Ld_Final*/1 -> Resettable Delay/3
  U_delay/1 -> Resettable Delay1/3
  r(k-1)/1 -> Ld_Final**/1
  Ld_Final**/1 -> Resettable Delay2/3
  Initial Velocities/1 -> VH2P/4(Iintial Velocities)
  Initial HeadingAngles/1 -> VH2P/5(Iintial HeadingAngles)
  From Workspace2/1 -> gate/1(select_overlap)
  gate/1(state) -> Resettable Delay/2, Resettable Delay1/2, Resettable Delay2/2
  G_Final/1 -> Sum6/2

== system Copy_of_MPC_control/observer/simulator_5 ==
  r(k) : Inport
  r(k-1) : Inport  Port=2
  Initial position : Inport  Port=3
  Initial Velocities : Inport  Port=4
  Initial HeadingAngles : Inport  Port=5
  U_delay : Inport  Port=6
  xhat : Inport  Port=7
  C_Brake : Gain  Gain=C_Brake  Multiplication=Matrix(K*u) (u vector)
  C_Brake* : Gain  Gain=C_Brake  Multiplication=Matrix(K*u) (u vector)
  C_out_Brake : Gain  Gain=C_out_Brake  Multiplication=Matrix(K*u) (u vector)
  D_out_Brake : Gain  Gain=D_out_Brake  Multiplication=Matrix(K*u) (u vector)
  Demux : Demux  Outputs=2
  From Workspace2 : FromWorkspace  VariableName=select_overlap  SampleTime=Ts
  G_Brake : Gain  Gain=G_Brake  Multiplication=Matrix(K*u) (u vector)
  G_sys_Brake : Gain  Gain=G_sys_Brake  Multiplication=Matrix(K*u) (u vector)
  H_Brake : Gain  Gain=H_Brake  Multiplication=Matrix(K*u) (u vector)
  H_sys_Brake : Gain  Gain=H_sys_Brake  Multiplication=Matrix(K*u) (u vector)
  Ld_Brake : Gain  Gain=Ld_Brake  Multiplication=Matrix(K*u) (u vector)
  Ld_Brake* : Gain  Gain=Ld_Brake  Multiplication=Matrix(K*u) (u vector)
  Ld_Brake** : Gain  Gain=Ld_Brake  Multiplication=Matrix(K*u) (u vector)
  Mpc_Simulator_Middle : Subsystem
  Resettable Delay : Delay  DelayLength=1  InitialConditionSource=Input port  ExternalReset=Rising  SampleTime=Ts
      settings: InputPortMap=u0,r5,p4
  Resettable Delay1 : Delay  DelayLength=1  InitialConditionSource=Input port  ExternalReset=Rising  SampleTime=Ts
      settings: InputPortMap=u0,r5,p4
  Resettable Delay2 : Delay  DelayLength=1  InitialConditionSource=Input port  ExternalReset=Rising  SampleTime=Ts
      settings: InputPortMap=u0,r5,p4
  Sum1 : Sum  Inputs=+++
  Sum2 : Sum  Inputs=+++
  Sum6 : Sum
  Sum7 : Sum  Inputs=-+
  VH2P : Subsystem
  YV_update_Np : Subsystem  TreatAsAtomicUnit=on
  gate : MATLAB Function  TreatAsAtomicUnit=on
  Y_overlap : Outport
  U_overlap : Outport  Port=2
  wires:
  Initial position/1 -> VH2P/3(Initial position)
  Sum2/1 -> Resettable Delay/1
  Demux/2 -> YV_update_Np/3(Heading_sim), VH2P/2(HeadingAngles)
  Ld_Brake/1 -> Sum2/1
  Sum7/1 -> Ld_Brake/1
  Mpc_Simulator_Middle/2(r) -> Sum7/2
  C_out_Brake/1 -> Sum1/3
  C_Brake*/1 -> Sum7/1
  Mpc_Simulator_Middle/1(U) -> Resettable Delay1/1, H_sys_Brake/1, H_Brake/1, U_overlap/1
  H_sys_Brake/1 -> Sum2/2
  G_sys_Brake/1 -> Sum2/3
  Resettable Delay2/1 -> C_out_Brake/1
  VH2P/1(Position) -> YV_update_Np/1(XY_sim)
  Demux/1 -> VH2P/1(Velocities), YV_update_Np/2(Velocity_sim)
  Resettable Delay/1 -> G_sys_Brake/1, Resettable Delay2/1, G_Brake/1, C_Brake/1
  H_Brake/1 -> Sum6/1
  Sum1/1 -> Demux/1, Y_overlap/1
  Sum6/1 -> C_Brake*/1
  D_out_Brake/1 -> Sum1/2
  Resettable Delay1/1 -> D_out_Brake/1
  C_Brake/1 -> Sum1/1
  YV_update_Np/2(Heading_updated) -> Mpc_Simulator_Middle/2(Heading_updated)
  xhat/1 -> Mpc_Simulator_Middle/3(Xhat)
  YV_update_Np/1(Velocity_updated) -> Mpc_Simulator_Middle/1(Velocity_updated)
  r(k)/1 -> Ld_Brake*/1
  Ld_Brake*/1 -> Resettable Delay/3
  U_delay/1 -> Resettable Delay1/3
  r(k-1)/1 -> Ld_Brake**/1
  Ld_Brake**/1 -> Resettable Delay2/3
  Initial Velocities/1 -> VH2P/4(Iintial Velocities)
  Initial HeadingAngles/1 -> VH2P/5(Iintial HeadingAngles)
  From Workspace2/1 -> gate/1(select_overlap)
  gate/1(state) -> Resettable Delay/2, Resettable Delay1/2, Resettable Delay2/2
  G_Brake/1 -> Sum6/2

== system Copy_of_MPC_control/observer123/Final Observer2 ==
  Final_switch : Inport
  U : Inport  Port=2
  Y : Inport  Port=3
  Rs : Inport  Port=4
  U_delay : Inport  Port=5
  r(k-1) : Inport  Port=6
  r(k) : Inport  Port=7
  Initial position : Inport  Port=8
  Initial Velocities : Inport  Port=9
  Initial HeadingAngles : Inport  Port=10
  Tsim : Inport  Port=11
  LastTsim : Inport  Port=12
  Enable : EnablePort
  C_Final2 : Gain  Gain=C_Final  Multiplication=Matrix(K*u) (u vector)
  Clock : Clock
  Clock1 : Clock
  Delay : Delay  DelayLength=1  InitialConditionSource=Input port  InitialCondition=0  ExternalReset=Falling  SampleTime=Ts
      settings: InputPortMap=u0,r5,p4
  Delay1 : Delay  DelayLength=1  InitialConditionSource=Input port  InitialCondition=0  ExternalReset=Falling  SampleTime=Ts
      settings: InputPortMap=u0,r5,p4
  Final_switch3 : InportShadow
  Final_switch4 : InportShadow
  Gd_Final : Gain  Gain=Gd_Final  Multiplication=Matrix(K*u) (u vector)
  Hd_Final : Gain  Gain=Hd_Final  Multiplication=Matrix(K*u) (u vector)
  Ld_Final1 : Gain  Gain=Ld_Final  Multiplication=Matrix(K*u) (u vector)
  Ld_Final2 : Gain  Gain=Ld_Final  Multiplication=Matrix(K*u) (u vector)
  Subsystem : Subsystem
  Sum4 : Sum  Inputs=+++
  Switch : Switch  Threshold=Timetochange2
  Switch1 : Switch  Threshold=Timetochange2
  To Workspace : ToWorkspace  VariableName=FW  SaveFormat=Timeseries  SampleTime=Ts
  yhat : Outport
  xhat_delay : Outport  Port=2
  u_delay : Outport  Port=3
  xhat : Outport  Port=4
  wires:
  Switch/1 -> Delay1/1
  U/1 -> Switch/1
  Gd_Final/1 -> Sum4/3
  Delay/1 -> Gd_Final/1, xhat_delay/1
  Ld_Final1/1 -> Sum4/1
  Hd_Final/1 -> Sum4/2
  C_Final2/1 -> yhat/1
  Delay1/1 -> u_delay/1, Hd_Final/1
  Sum4/1 -> Subsystem/11(Xh_sim), xhat/1, C_Final2/1, Delay/1
  Y/1 -> Switch1/1
  Switch1/1 -> Ld_Final1/1
  r(k-1)/1 -> Ld_Final2/1, Subsystem/9(r(k-1))
  Ld_Final2/1 -> Delay/3
  r(k)/1 -> Subsystem/10(r(k))
  Rs/1 -> Subsystem/2(Rs)
  U_delay/1 -> Delay1/3, Subsystem/3(U_delay)
  Initial position/1 -> Subsystem/4(Initial position)
  Initial Velocities/1 -> Subsystem/5(Initial Velocities)
  Initial HeadingAngles/1 -> Subsystem/6(Initial HeadingAngles)
  Tsim/1 -> Subsystem/7(Tsim)
  LastTsim/1 -> Subsystem/8(LastTsim)
  Subsystem/1(Y) -> Switch1/3
  Subsystem/2(U) -> Switch/3
  Final_switch/1 -> To Workspace/1, Subsystem/1(Initial trigger)
  Final_switch3/1 -> Delay1/2
  Final_switch4/1 -> Delay/2
  Clock/1 -> Switch/2
  Clock1/1 -> Switch1/2

== system Copy_of_MPC_control/observer123/Front Observer2 ==
  Y : Inport
  U : Inport  Port=2
  Enable : EnablePort
  Cso : Gain  Gain=Cso  Multiplication=Matrix(K*u) (u vector)
  "Gsd " : Gain  Gain=Gsd  Multiplication=Matrix(K*u) (u vector)
  Hsd : Gain  Gain=Hsd  Multiplication=Matrix(K*u) (u vector)
  Lsd : Gain  Gain=Lsd  Multiplication=Matrix(K*u) (u vector)
  Sum3 : Sum  Inputs=+++
  Unit Delay2 : UnitDelay  InitialCondition=xho  SampleTime=Ts
  Unit Delay3 : UnitDelay  InitialCondition=[0;0]  SampleTime=Ts
  yhat : Outport
  xhat_delay : Outport  Port=2
  u_delay : Outport  Port=3
  xhat : Outport  Port=4
  wires:
  Unit Delay3/1 -> u_delay/1, Hsd/1
  "Gsd "/1 -> Sum3/3
  Lsd/1 -> Sum3/1
  Unit Delay2/1 -> xhat_delay/1, "Gsd "/1
  U/1 -> Unit Delay3/1
  Hsd/1 -> Sum3/2
  Y/1 -> Lsd/1
  Cso/1 -> yhat/1
  Sum3/1 -> xhat/1, Cso/1, Unit Delay2/1

== system Copy_of_MPC_control/observer123/Middle Observer2 ==
  U : Inport
  Y : Inport  Port=2
  Rs : Inport  Port=3
  Initial position : Inport  Port=4
  U_delay : Inport  Port=5
  r(k-1) : Inport  Port=6
  r(k) : Inport  Port=7
  Initial Velocities : Inport  Port=8
  Initial HeadingAngles : Inport  Port=9
  Tsim : Inport  Port=10
  LastTsim : Inport  Port=11
  Enable : EnablePort
  Clock : Clock
  Clock1 : Clock
  Co : Gain  Gain=Co  Multiplication=Matrix(K*u) (u vector)
  Delay : Delay  DelayLength=1  InitialConditionSource=Input port  InitialCondition=0  SampleTime=Ts
      settings: InputPortMap=u0,p4
  Delay1 : Delay  DelayLength=1  InitialConditionSource=Input port  InitialCondition=0  SampleTime=Ts
      settings: InputPortMap=u0,p4
  Gd : Gain  Gain=Gd  Multiplication=Matrix(K*u) (u vector)
  Hd : Gain  Gain=Hd  Multiplication=Matrix(K*u) (u vector)
  Ld : Gain  Gain=Ld  Multiplication=Matrix(K*u) (u vector)
  Ld1 : Gain  Gain=Ld  Multiplication=Matrix(K*u) (u vector)
  Observer_state2 : Subsystem
  Subsystem : Subsystem
  Sum4 : Sum  Inputs=+++
  Switch : Switch  Threshold=Timetochange
  Switch1 : Switch  Threshold=Timetochange
  yhat : Outport
  xhat_delay : Outport  Port=2
  u_delay : Outport  Port=3
  xhat : Outport  Port=4
  wires:
  Delay1/1 -> u_delay/1, Hd/1
  Sum4/1 -> xhat/1, Subsystem/10(xhat), Co/1, Delay/1
  Co/1 -> yhat/1
  Hd/1 -> Sum4/2
  Gd/1 -> Sum4/3
  Ld/1 -> Sum4/1
  Delay/1 -> Gd/1, xhat_delay/1
  U/1 -> Switch/1
  Switch/1 -> Delay1/1
  Ld1/1 -> Delay/2
  Y/1 -> Switch1/1
  Switch1/1 -> Ld/1
  Clock/1 -> Switch/2
  Clock1/1 -> Switch1/2
  Rs/1 -> Subsystem/1(Rs)
  Initial position/1 -> Subsystem/5(Initial position)
  Subsystem/2(U) -> Switch/3
  Observer_state2/1(state) -> Subsystem/Enable
  Subsystem/1(Y) -> Switch1/3
  r(k-1)/1 -> Ld1/1, Subsystem/4(r(k-1))
  U_delay/1 -> Delay1/2, Subsystem/2(U_delay)
  r(k)/1 -> Subsystem/3(r(k))
  Initial Velocities/1 -> Subsystem/6(Initial Velocities)
  Initial HeadingAngles/1 -> Subsystem/7(Initial HeadingAngles)
  Tsim/1 -> Subsystem/8(Tsim)
  LastTsim/1 -> Subsystem/9(LastTsim)

== system Copy_of_MPC_control/observer123/Observer_state1 ==
  Clock9 : Clock
  Observer_state1 : MATLAB Function  TreatAsAtomicUnit=on  SystemSampleTime=Ts
  Timetochange : Constant  Value=Timetochange  VectorParams1D=off  SampleTime=-1
  state : Outport
  wires:
  Timetochange/1 -> Observer_state1/2(point)
  Clock9/1 -> Observer_state1/1(timing)
  Observer_state1/1(state) -> state/1

== system Copy_of_MPC_control/observer123/Observer_state2 ==
  Clock9 : Clock
  Observer_state2 : MATLAB Function  TreatAsAtomicUnit=on  SystemSampleTime=Ts
  Timetochange : Constant  Value=Earlytochange  VectorParams1D=off  SampleTime=-1
  Timetochange1 : Constant  Value=Timetochange2  VectorParams1D=off  SampleTime=-1
  state : Outport
  wires:
  Timetochange/1 -> Observer_state2/2(Earlytochange)
  Clock9/1 -> Observer_state2/1(timing)
  Observer_state2/1(state) -> state/1
  Timetochange1/1 -> Observer_state2/3(Timetochange2)

== system Copy_of_MPC_control/observer123/Observer_state3 ==
  Clock9 : Clock
  Observer_state2 : MATLAB Function  TreatAsAtomicUnit=on  SystemSampleTime=Ts
  Timetochange : Constant  Value=Earlytochange2  VectorParams1D=off  SampleTime=-1
  state : Outport
  wires:
  Timetochange/1 -> Observer_state2/2(Earlytochange2)
  Clock9/1 -> Observer_state2/1(timing)
  Observer_state2/1(state) -> state/1

== system Copy_of_MPC_control/observer123/Select_model1 ==
  Clock14 : Clock
  Constant2 : Constant  Value=Timetochange2
  Constant3 : Constant  Value=Timetochange
  Select_model : MATLAB Function  TreatAsAtomicUnit=on  SystemSampleTime=Ts
  Select : Outport
  wires:
  Constant3/1 -> Select_model/2(Tc1)
  Constant2/1 -> Select_model/3(Tc2)
  Clock14/1 -> Select_model/1(Time)
  Select_model/1(Select) -> Select/1

== system Copy_of_MPC_control/Controllers/Brake Controller/Brake Pressure Control ==
  note: 1) Add Subsystem or Model blocks as valid variant choices.
      | 2) You cannot connect blocks at this level. At simulation, connectivity is automatically
      | determined, based on the active variant and port name matching.
  Pref : Inport
  xdot : Inport  Port=2
  <Kappa> : Inport  Port=3
  Bang Bang ABS : Subsystem  VariantControl=1
  Open Loop : Subsystem  VariantControl=0
  PCmd : Outport

== system Copy_of_MPC_control/Controllers/Transmission Controller/TCM ==
  AccCmd : Inport
  EngSpd : Inport  Port=2
  VehSpdFdbk : Inport  Port=3
  function : TriggerPort  TriggerType=function-call  VariantControl=Variant
  Neutral Select : Subsystem
  Prop Shaft Speed LPF : DiscreteTransferFcn  Numerator=[0.000000000000000 0.009950166250832 ]  Denominator=[1.000000000000000 -0.990049833749168 ]  mask(DiscretizedDiscreteTransferFcn){}
      mask init:
      | %zoh
  TCM Shift Controller : Stateflow chart  TreatAsAtomicUnit=on
  prop speed to vehicle speed : Gain  Gain=0.45
  Gear Select : Outport
  wires:
  VehSpdFdbk/1 -> Prop Shaft Speed LPF/1
  TCM Shift Controller/1(GearState) -> Gear Select/1  "GearCmd"
  AccCmd/1 -> Neutral Select/1(AccCmd), TCM Shift Controller/2(pedal)  "AccCmd"
  Neutral Select/1(Neutral Select) -> TCM Shift Controller/3(Neutral)
  EngSpd/1 -> Neutral Select/2(EngSpd)
  prop speed to vehicle speed/1 -> TCM Shift Controller/1(speed)
  Prop Shaft Speed LPF/1 -> prop speed to vehicle speed/1
